simulink model "Simulation"  (R2018b)
settings: Solver=VariableStepAuto  StartTime=0.0  StopTime=10.0  RelTol=1e-3
undefined symbols (not defined in the file or in its folder): ae0, ae1, ae2, ae3, as0, as1, as2, as3, be1, g, Js, Jxy, L, La, masseP, masseS, R, r_abc, Rs, XA, XB, XC, YA, YB, YC
settings Model: Creator=Vincent  LastModifiedBy=Vincent

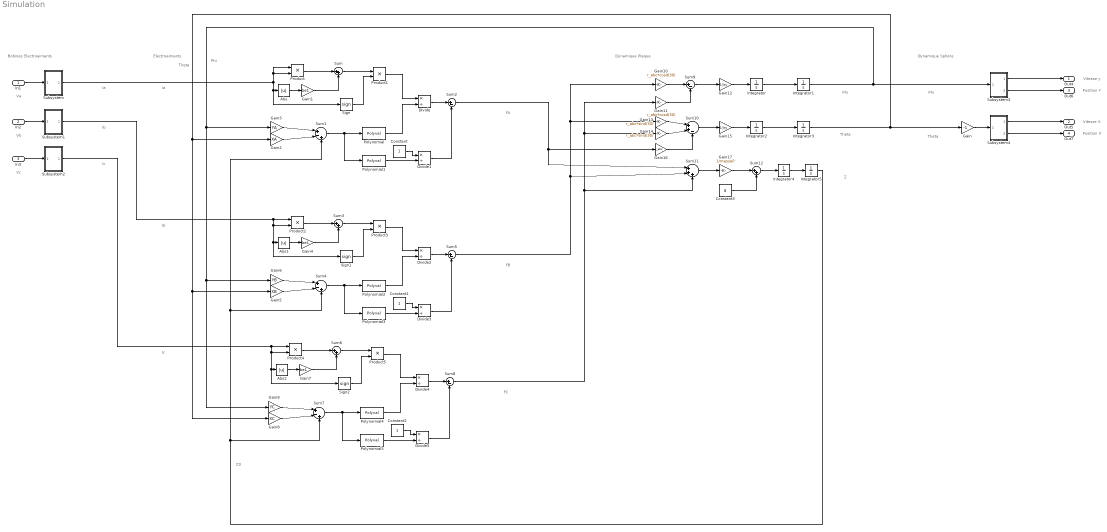
== system Simulation ==
  note: Z
  note: Ic
  note: Ib
  note: Ia
  note: Ic
  note: Ib
  note: Ia
  note: Theta
  note: Phi
  note: Vc
  note: Vb
  note: Va
  note: Z0
  note: FA
  note: Phi
  note: Theta
  note: Position X
  note: Vitesse X
  note: Position Y
  note: Vitesse y
  note: Phi
  note: Dynamique Sphère
  note: Dynamique Plaque
  note: Électroaimants
  note: Bobines Electroaimants
  note: Theta
  note: FB
  note: FC
  In1 : Inport
  In2 : Inport  Port=2
  In3 : Inport  Port=3
  Abs : Abs
  Abs1 : Abs
  Abs2 : Abs
  Constant : Constant
  Constant1 : Constant
  Constant2 : Constant
  Constant3 : Constant  Value=g
  Divide{,1..5} (6 alike) : Product  Inputs=*/
  Gain : Gain  Gain=-1
  Gain1 : Gain  Gain=be1
  Gain10 : Gain  Gain=r_abc*cosd(30)
  Gain11 : Gain  Gain=r_abc*cosd(30)
  Gain12 : Gain  Gain=1/Jxy
  Gain13 : Gain  Gain=r_abc*sind(30)
  Gain14 : Gain  Gain=r_abc*sind(30)
  Gain15 : Gain  Gain=1/Jxy
  Gain16 : Gain  Gain=r_abc
  Gain17 : Gain  Gain=1/masseP
  Gain2 : Gain  Gain=XA
  Gain3 : Gain  Gain=YA
  Gain4 : Gain  Gain=be1
  Gain5 : Gain  Gain=XB
  Gain6 : Gain  Gain=YB
  Gain7 : Gain  Gain=be1
  Gain8 : Gain  Gain=XC
  Gain9 : Gain  Gain=YC
  Integrator{,1..5} (6 alike) : Integrator
  Polynomial : Polyval  Coefs=[ae3 ae2 ae1 ae0]
  Polynomial1 : Polyval  Coefs=[as3 as2 as1 as0]
  Polynomial2 : Polyval  Coefs=[ae3 ae2 ae1 ae0]
  Polynomial3 : Polyval  Coefs=[as3 as2 as1 as0]
  Polynomial4 : Polyval  Coefs=[ae3 ae2 ae1 ae0]
  Polynomial5 : Polyval  Coefs=[as3 as2 as1 as0]
  Product{,1..5} (6 alike) : Product
  Sign : Signum
  Sign1 : Signum
  Sign2 : Signum
  Subsystem : Subsystem
  Subsystem1 : Subsystem
  Subsystem2 : Subsystem
  Subsystem3 : Subsystem
  Subsystem4 : Subsystem
  Sum{,3,6,12} (4 alike) : Sum  Inputs=|++
  Sum1 : Sum  Inputs=|+-+
  Sum10 : Sum  Inputs=|++-
  Sum11 : Sum  Inputs=|+++
  Sum{2,5,8..9} (4 alike) : Sum  Inputs=|+-
  Sum4 : Sum  Inputs=|+-+
  Sum7 : Sum  Inputs=|+-+
  Out4 : Outport
  Out5 : Outport  Port=2
  Out6 : Outport  Port=3
  Out7 : Outport  Port=4
  wires:
  In1/1 -> Subsystem/1(In1)
  In2/1 -> Subsystem1/1(In1)
  In3/1 -> Subsystem2/1(In1)
  Subsystem3/1(Out4) -> Out4/1
  Subsystem4/1(Out4) -> Out5/1
  Gain/1 -> Subsystem4/1(In4)
  Subsystem3/2(Out1) -> Out6/1
  Subsystem4/2(Out1) -> Out7/1
  Integrator/1 -> Integrator1/1
  Abs/1 -> Gain1/1
  Subsystem/1(Out1) -> Product/1, Product/2, Abs/1, Sign/1
  Product/1 -> Sum/1
  Gain1/1 -> Sum/2
  Sum/1 -> Product1/1
  Sign/1 -> Product1/2
  Product1/1 -> Divide/1
  Polynomial/1 -> Divide/2
  Integrator1/1 -> Gain9/1, Gain6/1, Gain3/1, Subsystem3/1(In4)
  Integrator3/1 -> Gain/1, Gain8/1, Gain5/1, Gain2/1
  Gain2/1 -> Sum1/2
  Gain3/1 -> Sum1/1
  Sum1/1 -> Polynomial1/1, Polynomial/1
  Divide/1 -> Sum2/1
  Polynomial1/1 -> Divide1/2
  Constant/1 -> Divide1/1
  Divide1/1 -> Sum2/2
  Constant1/1 -> Divide3/1
  Divide3/1 -> Sum5/2
  Gain6/1 -> Sum4/1
  Divide2/1 -> Sum5/1
  Sign1/1 -> Product3/2
  Sum4/1 -> Polynomial3/1, Polynomial2/1
  Gain5/1 -> Sum4/2
  Polynomial3/1 -> Divide3/2
  Subsystem1/1(Out1) -> Product2/1, Abs1/1, Sign1/1, Product2/2
  Gain4/1 -> Sum3/2
  Product3/1 -> Divide2/1
  Abs1/1 -> Gain4/1
  Product2/1 -> Sum3/1
  Polynomial2/1 -> Divide2/2
  Sum3/1 -> Product3/1
  Constant2/1 -> Divide5/1
  Divide5/1 -> Sum8/2
  Gain9/1 -> Sum7/1
  Divide4/1 -> Sum8/1
  Sign2/1 -> Product5/2
  Sum7/1 -> Polynomial5/1, Polynomial4/1
  Gain8/1 -> Sum7/2
  Polynomial5/1 -> Divide5/2
  Subsystem2/1(Out1) -> Abs2/1, Sign2/1, Product4/2, Product4/1
  Gain7/1 -> Sum6/2
  Product5/1 -> Divide4/1
  Abs2/1 -> Gain7/1
  Product4/1 -> Sum6/1
  Polynomial4/1 -> Divide4/2
  Sum6/1 -> Product5/1
  Integrator5/1 -> Sum1/3, Sum4/3, Sum7/3
  Sum9/1 -> Gain12/1
  Gain12/1 -> Integrator/1
  Gain10/1 -> Sum9/1
  Gain11/1 -> Sum9/2
  Gain15/1 -> Integrator2/1
  Gain14/1 -> Sum10/2
  Sum10/1 -> Gain15/1
  Integrator2/1 -> Integrator3/1
  Gain13/1 -> Sum10/1
  Gain16/1 -> Sum10/3
  Sum8/1 -> Sum11/3, Gain14/1, Gain11/1
  Sum2/1 -> Sum11/1, Gain16/1
  Sum5/1 -> Sum11/2, Gain13/1, Gain10/1
  Sum11/1 -> Gain17/1
  Gain17/1 -> Sum12/1
  Constant3/1 -> Sum12/2
  Sum12/1 -> Integrator4/1
  Integrator4/1 -> Integrator5/1

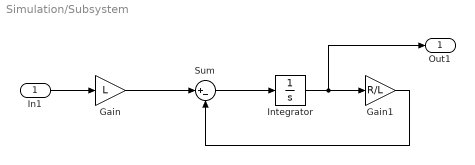
== system Simulation/Subsystem ==
  In1 : Inport
  Gain : Gain  Gain=L
  Gain1 : Gain  Gain=R/L
  Integrator : Integrator
  Sum : Sum  Inputs=|+-
  Out1 : Outport
  wires:
  Integrator/1 -> Out1/1, Gain1/1
  Gain/1 -> Sum/1
  Gain1/1 -> Sum/2
  Sum/1 -> Integrator/1
  In1/1 -> Gain/1

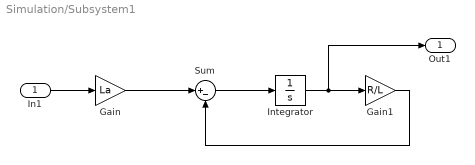
== system Simulation/Subsystem1 ==
  In1 : Inport
  Gain : Gain  Gain=La
  Gain1 : Gain  Gain=R/L
  Integrator : Integrator
  Sum : Sum  Inputs=|+-
  Out1 : Outport
  wires:
  Integrator/1 -> Out1/1, Gain1/1
  Gain/1 -> Sum/1
  Gain1/1 -> Sum/2
  Sum/1 -> Integrator/1
  In1/1 -> Gain/1

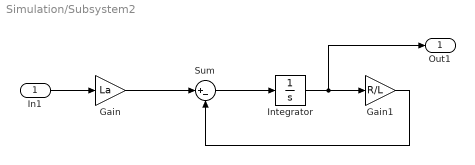
== system Simulation/Subsystem2 ==
  In1 : Inport
  Gain : Gain  Gain=La
  Gain1 : Gain  Gain=R/L
  Integrator : Integrator
  Sum : Sum  Inputs=|+-
  Out1 : Outport
  wires:
  Integrator/1 -> Out1/1, Gain1/1
  Gain/1 -> Sum/1
  Gain1/1 -> Sum/2
  Sum/1 -> Integrator/1
  In1/1 -> Gain/1

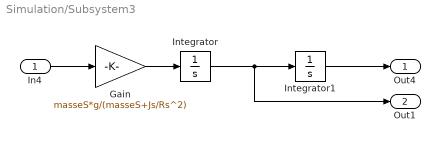
== system Simulation/Subsystem3 ==
  In4 : Inport  Tag=Theta
  Gain : Gain  Gain=masseS*g/(masseS+Js/Rs^2)
  Integrator : Integrator
  Integrator1 : Integrator
  Out4 : Outport
  Out1 : Outport  Port=2
  wires:
  Gain/1 -> Integrator/1
  In4/1 -> Gain/1
  Integrator1/1 -> Out4/1
  Integrator/1 -> Out1/1, Integrator1/1

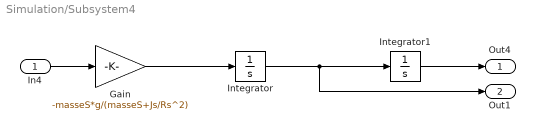
== system Simulation/Subsystem4 ==
  In4 : Inport  Tag=Theta
  Gain : Gain  Gain=-masseS*g/(masseS+Js/Rs^2)
  Integrator : Integrator
  Integrator1 : Integrator
  Out4 : Outport
  Out1 : Outport  Port=2
  wires:
  Gain/1 -> Integrator/1
  In4/1 -> Gain/1
  Integrator1/1 -> Out4/1
  Integrator/1 -> Out1/1, Integrator1/1
